simulink model "fazi_kontroleri"  (R2021a)
settings: Solver=VariableStepAuto  StartTime=0.0  StopTime=1000  RelTol=1e-3
libraries: fuzblock x5
settings Model: Creator=PC  LastModifiedBy=Maja

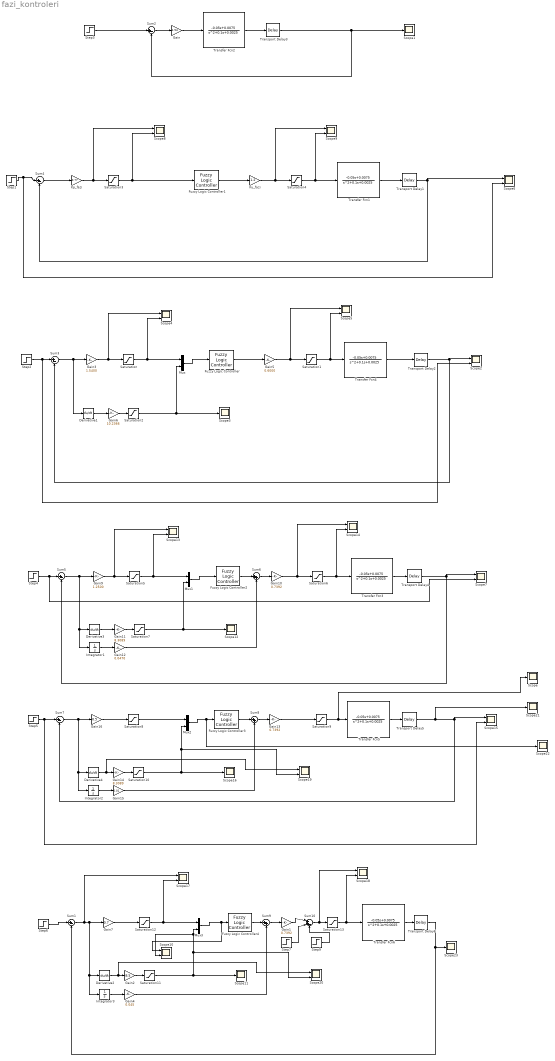
== system fazi_kontroleri ==
  Derivative{1..4} (4 alike) : Derivative
  Fuzzy Logic Controller : fuzblock/Fuzzy Logic  Controller  FIS='PDregulator.fis'  OutputSampleNumber=101  DataType=double  FuzzifiedInputs=off  RuleFiringStrengths=off  RuleOutputs=off  AggregatedOutputs=off  SimulateUsing=Interpreted execution  OutOfRangeInputValueMessage=warning  NoRuleFiredMessage=warning  EmptyOutputFuzzySetMessage=warning
  Fuzzy Logic Controller1 : fuzblock/Fuzzy Logic  Controller  FIS='Pregulator.fis'  OutputSampleNumber=101  DataType=double  FuzzifiedInputs=off  RuleFiringStrengths=off  RuleOutputs=off  AggregatedOutputs=off  SimulateUsing=Interpreted execution  OutOfRangeInputValueMessage=warning  NoRuleFiredMessage=warning  EmptyOutputFuzzySetMessage=warning
  Fuzzy Logic Controller2 : fuzblock/Fuzzy Logic  Controller  FIS='PDregulator.fis'  OutputSampleNumber=101  DataType=double  FuzzifiedInputs=off  RuleFiringStrengths=off  RuleOutputs=off  AggregatedOutputs=off  SimulateUsing=Interpreted execution  OutOfRangeInputValueMessage=warning  NoRuleFiredMessage=warning  EmptyOutputFuzzySetMessage=warning
  Fuzzy Logic Controller3 : fuzblock/Fuzzy Logic  Controller  FIS='PDnelinearan.fis'  OutputSampleNumber=101  DataType=double  FuzzifiedInputs=off  RuleFiringStrengths=off  RuleOutputs=off  AggregatedOutputs=off  SimulateUsing=Interpreted execution  OutOfRangeInputValueMessage=warning  NoRuleFiredMessage=warning  EmptyOutputFuzzySetMessage=warning
  Fuzzy Logic Controller4 : fuzblock/Fuzzy Logic  Controller  FIS='PDnelinearan.fis'  OutputSampleNumber=101  DataType=double  FuzzifiedInputs=off  RuleFiringStrengths=off  RuleOutputs=off  AggregatedOutputs=off  SimulateUsing=Interpreted execution  OutOfRangeInputValueMessage=warning  NoRuleFiredMessage=warning  EmptyOutputFuzzySetMessage=warning
  Gain : Gain  Gain=1.54
  Gain1 : Gain  Gain=0.7392
  Gain10 : Gain  Gain=0.7392
  Gain11 : Gain  Gain=8.3089
  Gain12 : Gain  Gain=0.0470
  Gain13 : Gain  Gain=0.7392
  Gain14 : Gain  Gain=8.3089
  Gain15 : Gain  Gain=0.01
  Gain16 : Gain  Gain=0.5
  Gain2 : Gain  Gain=8.5
  Gain3 : Gain  Gain=1.5400
  Gain4 : Gain  Gain=0.045
  Gain5 : Gain  Gain=0.6000
  Gain6 : Gain  Gain=10.2366
  Gain7 : Gain  Gain=0.7
  Gain9 : Gain  Gain=1.2500
  Integrator1 : Integrator
  Integrator2 : Integrator
  Integrator3 : Integrator
  Kp_fazi : Gain  Gain=0.77
  Ku_fazi : Gain  Gain=1.2
  Mux{,1..3} (4 alike) : Mux  Inputs=2
  Saturation{,2..3,5,7..8,10..12} (9 alike) : Saturate  UpperLimit=1  LowerLimit=-1
  Saturation{1,4,6,9,13} (5 alike) : Saturate  UpperLimit=1.2  LowerLimit=-1.2
  Scope{,1,3,11..12,16,21..23} (9 alike) : Scope
  Scope{2,4..10,13..15,17..20} (15 alike) : Scope  NumInputPorts=2
  Step{1..2,4..5} (4 alike) : Step  Time=500  Before=-2  After=2  SampleTime=0
  Step3 : Step  Time=50  SampleTime=0
  Step6 : Step  Time=10  After=0  SampleTime=0
  Step7 : Step  Time=10  After=0.6  SampleTime=0
  Step9 : Step  Time=500  After=0.6  SampleTime=0
  Sum{1..5,7} (6 alike) : Sum  Inputs=|+-
  Sum10 : Sum  Inputs=|++-
  Sum6 : Sum  Inputs=|++
  Sum8 : Sum  Inputs=|++
  Sum9 : Sum  Inputs=|++
  Transfer Fcn{1..6} (6 alike) : TransferFcn  Numerator=[-0.05 0.0075]  Denominator=[1 0.1 0.0025]
  Transport Delay{1..2,4..6} (5 alike) : TransportDelay  DelayTime=3.6
  Transport Delay3 : TransportDelay
  wires:
  Sum2/1 -> Gain/1
  Step3/1 -> Sum2/1
  Transport Delay3/1 -> Scope1/1, Sum2/2
  Transfer Fcn2/1 -> Transport Delay3/1
  Gain/1 -> Transfer Fcn2/1
  Saturation4/1 -> Transfer Fcn1/1, Scope9/2
  Transport Delay1/1 -> Sum4/2, Scope6/1
  Kp_fazi/1 -> Scope8/1, Saturation3/1
  Saturation3/1 -> Fuzzy Logic Controller1/1, Scope8/2
  Step1/1 -> Scope6/2, Sum4/1
  Sum4/1 -> Kp_fazi/1
  Ku_fazi/1 -> Scope9/1, Saturation4/1
  Fuzzy Logic Controller1/1 -> Ku_fazi/1
  Transfer Fcn1/1 -> Transport Delay1/1
  Mux/1 -> Fuzzy Logic Controller/1
  Gain6/1 -> Saturation2/1
  Saturation/1 -> Scope4/2, Mux/1
  Fuzzy Logic Controller/1 -> Gain5/1
  Transport Delay2/1 -> Sum3/2, Scope2/1
  Transfer Fcn4/1 -> Transport Delay2/1
  Derivative1/1 -> Gain6/1
  Gain5/1 -> Scope5/1, Saturation1/1
  Saturation2/1 -> Mux/2, Scope3/1
  Saturation1/1 -> Transfer Fcn4/1, Scope5/2
  Sum3/1 -> Derivative1/1, Gain3/1
  Gain3/1 -> Scope4/1, Saturation/1
  Gain11/1 -> Saturation7/1
  Saturation5/1 -> Scope13/2, Mux1/1
  Integrator1/1 -> Gain12/1
  Gain9/1 -> Scope13/1, Saturation5/1
  Step4/1 -> Scope7/2, Sum5/1
  Derivative3/1 -> Gain11/1
  Sum5/1 -> Integrator1/1, Derivative3/1, Gain9/1
  Gain10/1 -> Scope14/1, Saturation6/1
  Fuzzy Logic Controller2/1 -> Sum6/1
  Sum6/1 -> Gain10/1
  Mux1/1 -> Fuzzy Logic Controller2/1
  Saturation7/1 -> Mux1/2, Scope12/1
  Saturation6/1 -> Transfer Fcn3/1, Scope14/2
  Gain12/1 -> Sum6/2
  Transfer Fcn3/1 -> Transport Delay4/1
  Transport Delay4/1 -> Scope7/1, Sum5/2
  Integrator2/1 -> Gain15/1
  Transport Delay5/1 -> Scope21/1, Scope15/1, Sum7/2
  Gain14/1 -> Saturation10/1
  Derivative4/1 -> Scope19/1, Gain14/1
  Saturation8/1 -> Mux2/1
  Transfer Fcn5/1 -> Transport Delay5/1
  Sum7/1 -> Integrator2/1, Derivative4/1, Gain16/1
  Fuzzy Logic Controller3/1 -> Sum8/1
  Saturation10/1 -> Scope19/2, Mux2/2, Scope16/1
  Gain16/1 -> Saturation8/1
  Saturation9/1 -> Scope/1, Transfer Fcn5/1
  Gain15/1 -> Sum8/2
  Mux2/1 -> Scope22/1, Fuzzy Logic Controller3/1
  Sum8/1 -> Gain13/1
  Gain13/1 -> Saturation9/1
  Step5/1 -> Scope15/2, Sum7/1
  Gain1/1 -> Sum10/1
  Integrator3/1 -> Gain4/1
  Sum10/1 -> Scope18/1, Saturation13/1
  Transport Delay6/1 -> Sum1/2, Scope23/1
  Gain2/1 -> Saturation11/1
  Step9/1 -> Sum10/3
  Derivative2/1 -> Scope20/1, Gain2/1
  Step7/1 -> Sum10/2
  Saturation12/1 -> Scope17/2, Mux3/1
  Step6/1 -> Sum1/1
  Sum1/1 -> Scope17/1, Integrator3/1, Derivative2/1, Gain7/1
  Fuzzy Logic Controller4/1 -> Sum9/1
  Saturation11/1 -> Scope20/2, Mux3/2, Scope10/2, Scope11/1
  Gain7/1 -> Saturation12/1
  Saturation13/1 -> Transfer Fcn6/1, Scope18/2
  Gain4/1 -> Sum9/2
  Mux3/1 -> Scope10/1, Fuzzy Logic Controller4/1
  Sum9/1 -> Gain1/1
  Transfer Fcn6/1 -> Transport Delay6/1
  Step2/1 -> Scope2/2, Sum3/1
